simulink model "Md53StEnCtrl"  (R2018b)
settings: Solver=FixedStepDiscrete  StartTime=0.0  StopTime=10.0  FixedStep=0.01  RelTol=1e-3
undefined symbols (not defined in the file or in its folder): data, SecRwRtStBkReclnEn_Clear, SecRwRtStBkReclnEn_Set, ThdRwRtStBkReclnEn_Clear, ThdRwRtStBkReclnEn_Set, ThdRwRtStCshnFldEn_Clear, ThdRwRtStCshnFldEn_Set
libraries: simulink x1
settings Model: Creator=sn2xws  LastModifiedBy=sn2xws
settings Model: ModifiedHistory=|
  | 2024.6.24 V3.0.0 557模式流程V1.9
  | 2024.8.16 V3.0.1增加FirstTrig参数
  | 2024.8.20 V3.0.2 CshnFirstDone 时不调用电机
  | 2024.12.17 V3.0.3 BUG 962503 三排靠背与二排靠背应该一起动
settings DataIOCC: SaveFormat=StructureWithTime
settings OptimizationCC: DefaultParameterBehavior=Inlined  EnhancedBackFolding=on  PassReuseOutputArgsAs=Individual arguments  ZeroExternalMemoryAtStartup=off  ZeroInternalMemoryAtStartup=off  OptimizeBlockOrder=speed  DifferentSizesBufferReuse=on  OptimizationCustomize=off
settings DebuggingCC: ParameterTunabilityLossMsg=error
settings SFSimCC: MATLABDynamicMemAlloc=off
settings RTWCC: SystemTargetFile=autosar.tlc  GenCodeOnly=on  TemplateMakefile=ert_default_tmf  Description=AUTOSAR  GenerateReport=on  IncludeHyperlinkInReport=on  LaunchReport=on  GenerateTraceInfo=on  GenerateTraceReport=on  GenerateTraceReportSl=on  GenerateTraceReportSf=on  GenerateTraceReportEml=on
settings CodeAppCC: ForceParamTrailComments=on  IgnoreCustomStorageClasses=off  OperatorAnnotations=on  SimulinkDataObjDesc=on  SFDataObjDesc=on  InsertBlockDesc=on
settings STFCustomTargetCC: TargetLangStandard=C99 (ISO)  MultiwordLength=256  ParMdlRefBuildCompliant=on  CompOptLevelCompliant=on  IncludeMdlTerminateFcn=off  CombineOutputUpdateFcns=on  SuppressErrorStatus=on  ERTCustomFileBanners=on  SupportNonFinite=off  SupportComplex=off  SupportContinuousTime=off  SupportNonInlinedSFcns=off  RemoveResetFunc=on  MATLABClassNameForMDSCustomization=Simulink.SoftwareTarget.ERTCustomization  AutosarCompliant=on  UseToolchainInfoCompliant=on  LookupTableObjectStructAxisOrder=2,1,3,4,...  LUTObjectStructOrderEvenSpacing=Size,Table,Breakpoints  SystemTargetFile=autosar.tlc
settings ERTTargetCC: TargetLangStandard=C99 (ISO)  ConcurrentExecutionCompliant=off  IncludeMdlTerminateFcn=off  SuppressErrorStatus=on  SupportNonFinite=off  SupportComplex=off  ModelStepFunctionPrototypeControlCompliant=off  CPPClassGenCompliant=off  AutosarCompliant=on  LookupTableObjectStructAxisOrder=2,1,3,4,...  LUTObjectStructOrderEvenSpacing=Size,Table,Breakpoints  InlinedParameterPlacement=NonHierarchical  ERTCustomFileTemplate=example_file_process.tlc  ERTFilePackagingFormat=Compact

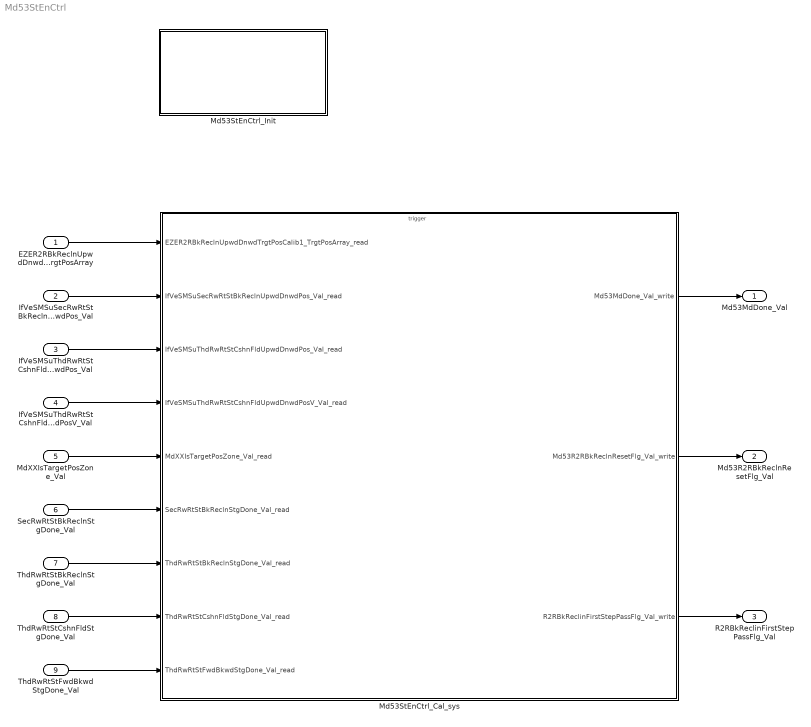
== system Md53StEnCtrl ==
  EZER2RBkReclnUpwdDnwdTrgtPosCalib1_TrgtPosArray : Inport  Description=|  OutDataTypeStr=uint16  PortDimensions=3
      | 0:Pos
      | 1:Max
      | 2:Min
  IfVeSMSuSecRwRtStBkReclnUpwdDnwdPos_Val : Inport  Port=2  OutDataTypeStr=uint16  PortDimensions=1
  IfVeSMSuThdRwRtStCshnFldUpwdDnwdPos_Val : Inport  Port=3  OutDataTypeStr=uint16  PortDimensions=1
  IfVeSMSuThdRwRtStCshnFldUpwdDnwdPosV_Val : Inport  Port=4  OutDataTypeStr=boolean  PortDimensions=1
  MdXXIsTargetPosZone_Val : Inport  Port=5  OutDataTypeStr=uint32  PortDimensions=1
  SecRwRtStBkReclnStgDone_Val : Inport  Port=6  OutDataTypeStr=boolean  PortDimensions=1
  ThdRwRtStBkReclnStgDone_Val : Inport  Port=7  OutDataTypeStr=boolean  PortDimensions=1
  ThdRwRtStCshnFldStgDone_Val : Inport  Port=8  OutDataTypeStr=boolean  PortDimensions=1
  ThdRwRtStFwdBkwdStgDone_Val : Inport  Port=9  OutDataTypeStr=boolean  PortDimensions=1
  Md53StEnCtrl_Cal_sys : Subsystem
  Md53StEnCtrl_Init : Subsystem
  Md53MdDone_Val : Outport  OutDataTypeStr=uint8  PortDimensions=1
  Md53R2RBkReclnResetFlg_Val : Outport  Port=2  OutDataTypeStr=boolean  PortDimensions=1
  R2RBkReclinFirstStepPassFlg_Val : Outport  Port=3  OutDataTypeStr=boolean  PortDimensions=1
  wires:
  EZER2RBkReclnUpwdDnwdTrgtPosCalib1_TrgtPosArray/1 -> Md53StEnCtrl_Cal_sys/1(EZER2RBkReclnUpwdDnwdTrgtPosCalib1_TrgtPosArray_read)
  IfVeSMSuSecRwRtStBkReclnUpwdDnwdPos_Val/1 -> Md53StEnCtrl_Cal_sys/2(IfVeSMSuSecRwRtStBkReclnUpwdDnwdPos_Val_read)
  IfVeSMSuThdRwRtStCshnFldUpwdDnwdPos_Val/1 -> Md53StEnCtrl_Cal_sys/3(IfVeSMSuThdRwRtStCshnFldUpwdDnwdPos_Val_read)
  IfVeSMSuThdRwRtStCshnFldUpwdDnwdPosV_Val/1 -> Md53StEnCtrl_Cal_sys/4(IfVeSMSuThdRwRtStCshnFldUpwdDnwdPosV_Val_read)
  MdXXIsTargetPosZone_Val/1 -> Md53StEnCtrl_Cal_sys/5(MdXXIsTargetPosZone_Val_read)
  SecRwRtStBkReclnStgDone_Val/1 -> Md53StEnCtrl_Cal_sys/6(SecRwRtStBkReclnStgDone_Val_read)
  ThdRwRtStBkReclnStgDone_Val/1 -> Md53StEnCtrl_Cal_sys/7(ThdRwRtStBkReclnStgDone_Val_read)
  ThdRwRtStCshnFldStgDone_Val/1 -> Md53StEnCtrl_Cal_sys/8(ThdRwRtStCshnFldStgDone_Val_read)
  ThdRwRtStFwdBkwdStgDone_Val/1 -> Md53StEnCtrl_Cal_sys/9(ThdRwRtStFwdBkwdStgDone_Val_read)
  Md53StEnCtrl_Cal_sys/1(Md53MdDone_Val_write) -> Md53MdDone_Val/1
  Md53StEnCtrl_Cal_sys/2(Md53R2RBkReclnResetFlg_Val_write) -> Md53R2RBkReclnResetFlg_Val/1
  Md53StEnCtrl_Cal_sys/3(R2RBkReclinFirstStepPassFlg_Val_write) -> R2RBkReclinFirstStepPassFlg_Val/1

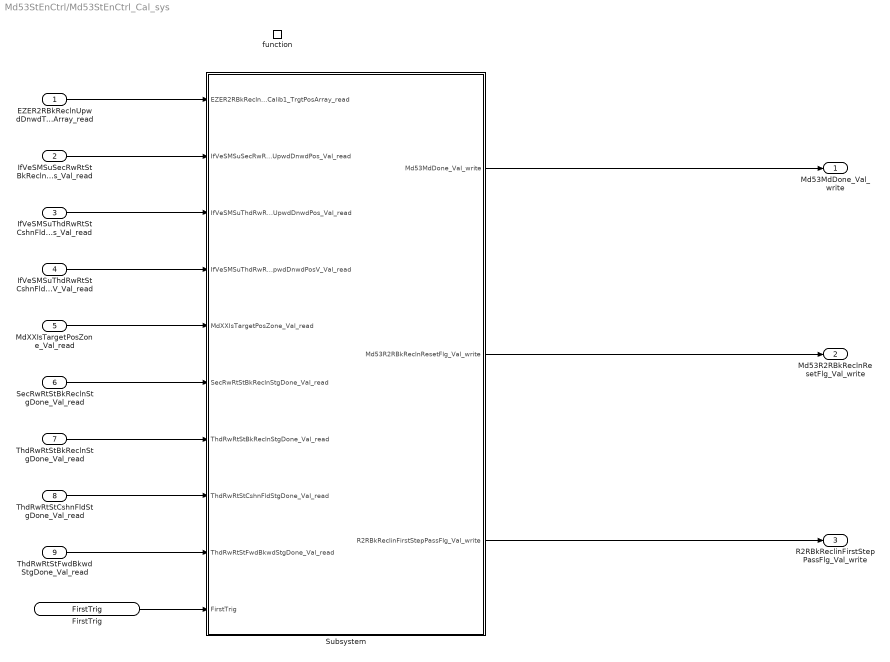
== system Md53StEnCtrl/Md53StEnCtrl_Cal_sys ==
  EZER2RBkReclnUpwdDnwdTrgtPosCalib1_TrgtPosArray_read : Inport
  IfVeSMSuSecRwRtStBkReclnUpwdDnwdPos_Val_read : Inport  Port=2
  IfVeSMSuThdRwRtStCshnFldUpwdDnwdPos_Val_read : Inport  Port=3
  IfVeSMSuThdRwRtStCshnFldUpwdDnwdPosV_Val_read : Inport  Port=4
  MdXXIsTargetPosZone_Val_read : Inport  Port=5
  SecRwRtStBkReclnStgDone_Val_read : Inport  Port=6
  ThdRwRtStBkReclnStgDone_Val_read : Inport  Port=7
  ThdRwRtStCshnFldStgDone_Val_read : Inport  Port=8
  ThdRwRtStFwdBkwdStgDone_Val_read : Inport  Port=9
  function : TriggerPort  TriggerType=function-call  IsSimulinkFunction=on  FunctionName=Md53StEnCtrl_Cal  VariantControl=(inherit)
  Subsystem : Subsystem
  FirstTrig : ArgIn  OutDataTypeStr=boolean  ArgumentName=FirstTrig
  Md53MdDone_Val_write : Outport
      settings: EnsureOutportIsVirtual=on
  Md53R2RBkReclnResetFlg_Val_write : Outport  Port=2
      settings: EnsureOutportIsVirtual=on
  R2RBkReclinFirstStepPassFlg_Val_write : Outport  Port=3
      settings: EnsureOutportIsVirtual=on
  wires:
  EZER2RBkReclnUpwdDnwdTrgtPosCalib1_TrgtPosArray_read/1 -> Subsystem/1(EZER2RBkReclnUpwdDnwdTrgtPosCalib1_TrgtPosArray_read)
  IfVeSMSuSecRwRtStBkReclnUpwdDnwdPos_Val_read/1 -> Subsystem/2(IfVeSMSuSecRwRtStBkReclnUpwdDnwdPos_Val_read)
  IfVeSMSuThdRwRtStCshnFldUpwdDnwdPos_Val_read/1 -> Subsystem/3(IfVeSMSuThdRwRtStCshnFldUpwdDnwdPos_Val_read)
  IfVeSMSuThdRwRtStCshnFldUpwdDnwdPosV_Val_read/1 -> Subsystem/4(IfVeSMSuThdRwRtStCshnFldUpwdDnwdPosV_Val_read)
  MdXXIsTargetPosZone_Val_read/1 -> Subsystem/5(MdXXIsTargetPosZone_Val_read)
  SecRwRtStBkReclnStgDone_Val_read/1 -> Subsystem/6(SecRwRtStBkReclnStgDone_Val_read)
  ThdRwRtStBkReclnStgDone_Val_read/1 -> Subsystem/7(ThdRwRtStBkReclnStgDone_Val_read)
  ThdRwRtStCshnFldStgDone_Val_read/1 -> Subsystem/8(ThdRwRtStCshnFldStgDone_Val_read)
  ThdRwRtStFwdBkwdStgDone_Val_read/1 -> Subsystem/9(ThdRwRtStFwdBkwdStgDone_Val_read)
  Subsystem/1(Md53MdDone_Val_write) -> Md53MdDone_Val_write/1
  Subsystem/2(Md53R2RBkReclnResetFlg_Val_write) -> Md53R2RBkReclnResetFlg_Val_write/1
  Subsystem/3(R2RBkReclinFirstStepPassFlg_Val_write) -> R2RBkReclinFirstStepPassFlg_Val_write/1
  FirstTrig/1 -> Subsystem/10(FirstTrig)

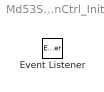
== system Md53StEnCtrl/Md53StEnCtrl_Init ==
  Event Listener : EventListener  EventName=reset

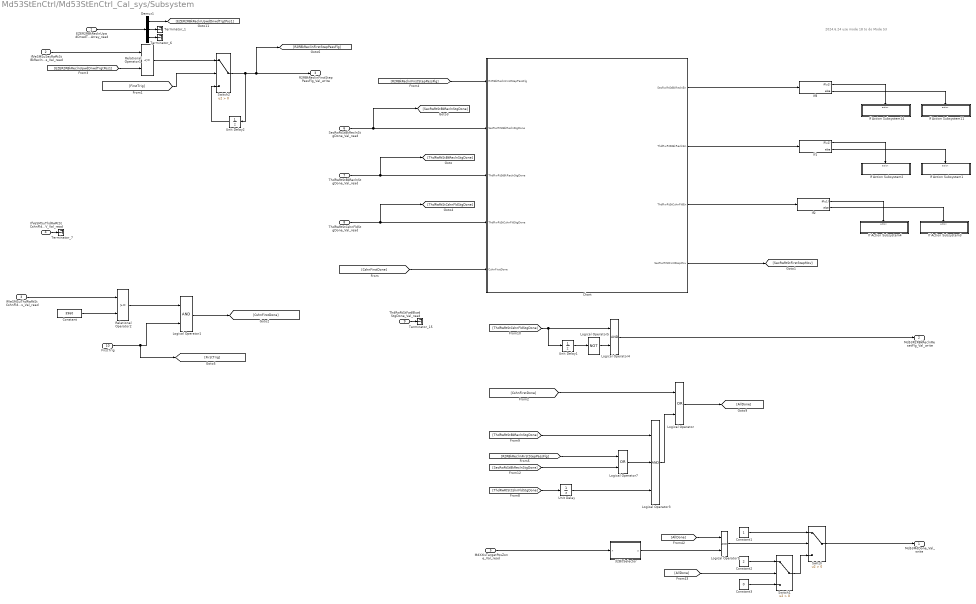
== system Md53StEnCtrl/Md53StEnCtrl_Cal_sys/Subsystem ==
  note: 2024.6.24 use mode 18 to do Mode 53
  EZER2RBkReclnUpwdDnwdTrgtPosCalib1_TrgtPosArray_read : Inport
  IfVeSMSuSecRwRtStBkReclnUpwdDnwdPos_Val_read : Inport  Port=2
  IfVeSMSuThdRwRtStCshnFldUpwdDnwdPos_Val_read : Inport  Port=3
  IfVeSMSuThdRwRtStCshnFldUpwdDnwdPosV_Val_read : Inport  Port=4
  MdXXIsTargetPosZone_Val_read : Inport  Port=5
  SecRwRtStBkReclnStgDone_Val_read : Inport  Port=6
  ThdRwRtStBkReclnStgDone_Val_read : Inport  Port=7
  ThdRwRtStCshnFldStgDone_Val_read : Inport  Port=8
  ThdRwRtStFwdBkwdStgDone_Val_read : Inport  Port=9
  FirstTrig : Inport  Port=10
  32BitSelector : Subsystem  mask(32 Bit Selector){BitNum=17}
      mask prompts: BitNum "Select Bit Number"
      mask help: Allows selection of a particular bit (0-31) out of a packed word up to 32 bits long. Output will be true if the bit number selected via the mask parameter is equal to one.
      mask TypeOptions BitNum: 0 | 1 | 2 | 3 | 4 | 5 | 6 | 7 | 8 | 9 | 10 | 11 | 12 | 13 | 14 | 15 | 16 | 17 | 18 | 19 | 20 | 21 | 22 | 23 | 24 | 25 | 26 | 27 | 28 | 29 | 30 | 31
      mask Display:
      | text(0.5, 0.8,'BIT','horizontalAlignment','center')
      | text(0.5, 0.5,'SELECTOR','horizontalAlignment','center')
      | text(0.5, 0.2,['-- Bit ',char(get_param(gcb,'BitNum')),' --'],'horizontalAlignment','center')
  Chart : Stateflow chart  TreatAsAtomicUnit=on
  Constant : Constant  Value=3960  OutDataTypeStr=uint16
  Constant1 : Constant  OutDataTypeStr=uint8
  Constant2 : Constant  Value=2  OutDataTypeStr=uint8
  Constant3 : Constant  Value=0  OutDataTypeStr=uint8
  Demux1 : Demux  Outputs=3
  If Action Subsystem1 : Subsystem  TreatAsAtomicUnit=on
  If Action Subsystem11 : Subsystem  TreatAsAtomicUnit=on
  If Action Subsystem14 : Subsystem  TreatAsAtomicUnit=on
  If Action Subsystem2 : Subsystem  TreatAsAtomicUnit=on
  If Action Subsystem3 : Subsystem  TreatAsAtomicUnit=on
  If Action Subsystem4 : Subsystem  TreatAsAtomicUnit=on
  If1 : If  IfExpression=u1
  If2 : If  IfExpression=u1
  If8 : If  IfExpression=u1
  Logical Operator : Logic  Operator=OR  AllPortsSameDT=off  OutDataTypeStr=boolean
  Logical Operator1 : Logic  AllPortsSameDT=off  OutDataTypeStr=boolean
  Logical Operator3 : Logic  Inputs=3  AllPortsSameDT=off  OutDataTypeStr=boolean
  Logical Operator4 : Logic  AllPortsSameDT=off  OutDataTypeStr=boolean
  Logical Operator5 : Logic  Operator=NOT  AllPortsSameDT=off  OutDataTypeStr=boolean
  Logical Operator7 : Logic  Operator=OR  AllPortsSameDT=off  OutDataTypeStr=boolean
  Logical Operator9 : Logic  AllPortsSameDT=off  OutDataTypeStr=boolean
  Relational Operator1 : RelationalOperator  Operator=<=  OutDataTypeStr=boolean  RndMeth=Simplest
  Relational Operator2 : RelationalOperator  OutDataTypeStr=boolean  RndMeth=Simplest
  Switch : Switch  Criteria=u2 > Threshold
  Switch1 : Switch  Criteria=u2 > Threshold
  Switch2 : Switch  Criteria=u2 > Threshold
  Terminator_{1,6..7,15} (4 alike) : Terminator
  Unit Delay : UnitDelay  SampleTime=-1
  Unit Delay1 : UnitDelay  SampleTime=-1
  Unit Delay2 : UnitDelay  SampleTime=-1
  Md53MdDone_Val_write : Outport
      settings: EnsureOutportIsVirtual=on
  Md53R2RBkReclnResetFlg_Val_write : Outport  Port=2
      settings: EnsureOutportIsVirtual=on
  R2RBkReclinFirstStepPassFlg_Val_write : Outport  Port=3
      settings: EnsureOutportIsVirtual=on
  wires:
  IfVeSMSuThdRwRtStCshnFldUpwdDnwdPosV_Val_read/1 -> Terminator_7/1
  ThdRwRtStCshnFldStgDone_Val_read/1 -> [ThdRwRtStCshnFldStgDone], Chart/4(ThdRwRtStCshnFldStgDone)
  ThdRwRtStBkReclnStgDone_Val_read/1 -> [ThdRwRtStBkReclnStgDone], Chart/3(ThdRwRtStBkReclnStgDone)
  ThdRwRtStFwdBkwdStgDone_Val_read/1 -> Terminator_15/1
  SecRwRtStBkReclnStgDone_Val_read/1 -> [SecRwRtStBkReclnStgDone], Chart/2(SecRwRtStBkReclnStgDone)
  Switch/1 -> Md53MdDone_Val_write/1
  Logical Operator4/1 -> Md53R2RBkReclnResetFlg_Val_write/1
  [AllDone] -> Logical Operator9/1
  Logical Operator9/1 -> Switch/2
  Switch1/1 -> Switch/3
  Constant1/1 -> Switch/1
  32BitSelector/1(y) -> Logical Operator9/2
  Constant2/1 -> Switch1/1
  [AllDone] -> Switch1/2
  MdXXIsTargetPosZone_Val_read/1 -> 32BitSelector/1(x)
  Constant3/1 -> Switch1/3
  [R2RBkReclinFirstStepPassFlg] -> Logical Operator7/1
  Logical Operator/1 -> [AllDone]
  [SecRwRtStBkReclnStgDone] -> Logical Operator7/2
  [ThdRwRtStBkReclnStgDone] -> Logical Operator3/1
  Logical Operator3/1 -> Logical Operator/2
  [ThdRwRtStCshnFldStgDone] -> Unit Delay/1
  Unit Delay/1 -> Logical Operator3/3
  Logical Operator7/1 -> Logical Operator3/2
  [CshnFirstDone] -> Logical Operator/1
  Logical Operator5/1 -> Logical Operator4/2
  [ThdRwRtStCshnFldStgDone] -> Unit Delay1/1, Logical Operator4/1
  Unit Delay1/1 -> Logical Operator5/1
  Constant/1 -> Relational Operator2/2
  IfVeSMSuThdRwRtStCshnFldUpwdDnwdPos_Val_read/1 -> Relational Operator2/1
  [CshnFirstDone] -> Chart/5(CshnFirstDone)
  Chart/4(SecRwRtStFirstStepMov) -> [SecRwRtStFirstStepMov]
  Demux1/1 -> [EZER2RBkReclnUpwdDnwdTrgtPos1]
  Demux1/3 -> Terminator_6/1
  Demux1/2 -> Terminator_1/1
  EZER2RBkReclnUpwdDnwdTrgtPosCalib1_TrgtPosArray_read/1 -> Demux1/1
  [EZER2RBkReclnUpwdDnwdTrgtPos1] -> Relational Operator1/2
  IfVeSMSuSecRwRtStBkReclnUpwdDnwdPos_Val_read/1 -> Relational Operator1/1
  Chart/1(SecRwRtStBkReclnEn) -> If8/1
  If8/2 -> If Action Subsystem11/Action
  If8/1 -> If Action Subsystem14/Action
  If1/1 -> If Action Subsystem2/Action
  If1/2 -> If Action Subsystem1/Action
  Chart/2(ThdRwRtStBkReclnEn) -> If1/1
  Chart/3(ThdRwRtStCshnFldEn) -> If2/1
  If2/2 -> If Action Subsystem3/Action
  If2/1 -> If Action Subsystem4/Action
  Logical Operator1/1 -> [CshnFirstDone]
  Relational Operator2/1 -> Logical Operator1/1
  FirstTrig/1 -> [FirstTrig], Logical Operator1/2
  [FirstTrig] -> Switch2/2
  Relational Operator1/1 -> Switch2/1
  Switch2/1 -> [R2RBkReclinFirstStepPassFlg], R2RBkReclinFirstStepPassFlg_Val_write/1, Unit Delay2/1
  Unit Delay2/1 -> Switch2/3
  [R2RBkReclinFirstStepPassFlg] -> Chart/1(R2RBkReclinFirstStepPassFlg)

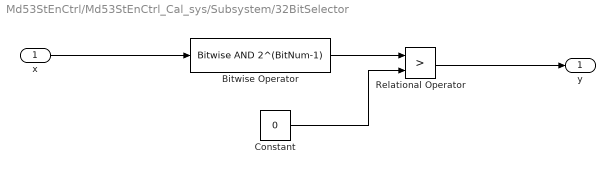
== system Md53StEnCtrl/Md53StEnCtrl_Cal_sys/Subsystem/32BitSelector ==
  x : Inport
  Bitwise Operator : simulink/Logic and Bit Operations/Bitwise Operator  logicop=AND  UseBitMask=on  BitMask=2^(BitNum-1)  BitMaskRealWorld=Stored Integer
  Constant : Constant  Value=0  OutDataTypeStr=uint32
  Relational Operator : RelationalOperator  Operator=>  OutDataTypeStr=boolean  RndMeth=Simplest
  y : Outport
  wires:
  Relational Operator/1 -> y/1
  Constant/1 -> Relational Operator/2
  x/1 -> Bitwise Operator/1
  Bitwise Operator/1 -> Relational Operator/1

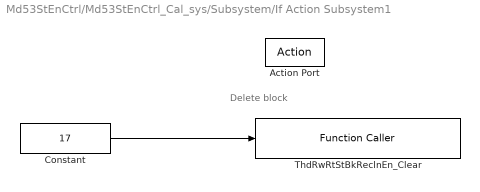
== system Md53StEnCtrl/Md53StEnCtrl_Cal_sys/Subsystem/If Action Subsystem1 ==
  note: Delete block
  Action Port : ActionPort  ActionType=else
  Constant : Constant  Value=17  OutDataTypeStr=uint8
  ThdRwRtStBkReclnEn_Clear : FunctionCaller  FunctionPrototype=ThdRwRtStBkReclnEn_Clear(data)  InputArgumentSpecifications=uint8(1)
  wires:
  Constant/1 -> ThdRwRtStBkReclnEn_Clear/1

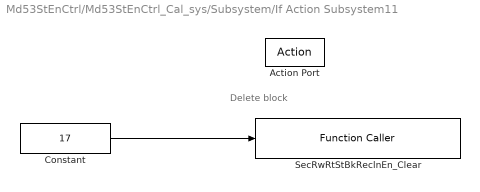
== system Md53StEnCtrl/Md53StEnCtrl_Cal_sys/Subsystem/If Action Subsystem11 ==
  note: Delete block
  Action Port : ActionPort  ActionType=else
  Constant : Constant  Value=17  OutDataTypeStr=uint8
  SecRwRtStBkReclnEn_Clear : FunctionCaller  FunctionPrototype=SecRwRtStBkReclnEn_Clear(data)  InputArgumentSpecifications=uint8(1)
  wires:
  Constant/1 -> SecRwRtStBkReclnEn_Clear/1

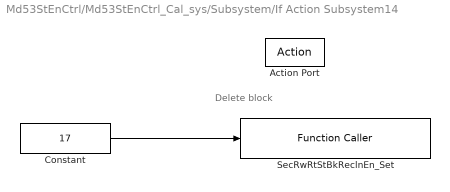
== system Md53StEnCtrl/Md53StEnCtrl_Cal_sys/Subsystem/If Action Subsystem14 ==
  note: Delete block
  Action Port : ActionPort  ActionType=then
  Constant : Constant  Value=17  OutDataTypeStr=uint8
  SecRwRtStBkReclnEn_Set : FunctionCaller  FunctionPrototype=SecRwRtStBkReclnEn_Set(data)  InputArgumentSpecifications=uint8(1)
  wires:
  Constant/1 -> SecRwRtStBkReclnEn_Set/1

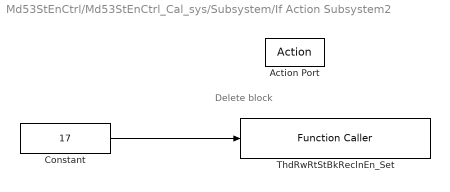
== system Md53StEnCtrl/Md53StEnCtrl_Cal_sys/Subsystem/If Action Subsystem2 ==
  note: Delete block
  Action Port : ActionPort  ActionType=then
  Constant : Constant  Value=17  OutDataTypeStr=uint8
  ThdRwRtStBkReclnEn_Set : FunctionCaller  FunctionPrototype=ThdRwRtStBkReclnEn_Set(data)  InputArgumentSpecifications=uint8(1)
  wires:
  Constant/1 -> ThdRwRtStBkReclnEn_Set/1

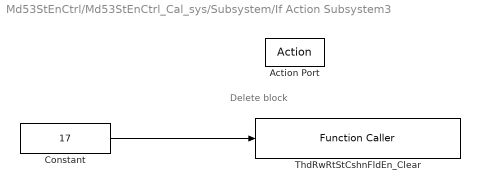
== system Md53StEnCtrl/Md53StEnCtrl_Cal_sys/Subsystem/If Action Subsystem3 ==
  note: Delete block
  Action Port : ActionPort  ActionType=else
  Constant : Constant  Value=17  OutDataTypeStr=uint8
  ThdRwRtStCshnFldEn_Clear : FunctionCaller  FunctionPrototype=ThdRwRtStCshnFldEn_Clear(data)  InputArgumentSpecifications=uint8(1)
  wires:
  Constant/1 -> ThdRwRtStCshnFldEn_Clear/1

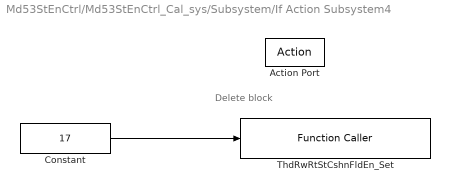
== system Md53StEnCtrl/Md53StEnCtrl_Cal_sys/Subsystem/If Action Subsystem4 ==
  note: Delete block
  Action Port : ActionPort  ActionType=then
  Constant : Constant  Value=17  OutDataTypeStr=uint8
  ThdRwRtStCshnFldEn_Set : FunctionCaller  FunctionPrototype=ThdRwRtStCshnFldEn_Set(data)  InputArgumentSpecifications=uint8(1)
  wires:
  Constant/1 -> ThdRwRtStCshnFldEn_Set/1

== stateflow chart Md53StEnCtrl/Md53StEnCtrl_Cal_sys/Subsystem/Chart ==
  (default) -> (junction 22) : {
      | SecRwRtStBkReclnEn = 0;
      | ThdRwRtStCshnFldEn = 0;
      | ThdRwRtStBkReclnEn = 0;
      | }
  (junction 22) -> (junction 83) [order 1] : [CshnFirstDone]
  (junction 22) -> (junction 25) [order 2]
  (junction 83) -> (junction 85)
  (junction 25) -> (junction 27) [order 1] : [R2RBkReclinFirstStepPassFlg ||SecRwRtStBkReclnStgDone]
  (junction 25) -> (junction 31) [order 2] : {
      | SecRwRtStBkReclnEn = 1;
      | }
  (junction 27) -> (junction 29)
  (junction 29) -> (junction 31)
  (junction 31) -> (junction 34)
  (junction 34) -> (junction 36) [order 1] : [(R2RBkReclinFirstStepPassFlg ||SecRwRtStBkReclnStgDone)]
  (junction 36) -> (junction 43) [order 1] : [ThdRwRtStCshnFldStgDone]
  (junction 34) -> (junction 75) [order 2]
  (junction 36) -> (junction 38) [order 2] : {ThdRwRtStCshnFldEn = 1;}
  (junction 43) -> (junction 66)
  (junction 38) -> (junction 75)
  (junction 66) -> (junction 38)
  (junction 75) -> (junction 78)
  (junction 78) -> (junction 94) [order 1] : [ThdRwRtStCshnFldStgDone]
  (junction 94) -> (junction 95) [order 1] : [ThdRwRtStBkReclnStgDone]
  (junction 78) -> (junction 97) [order 2]
  (junction 94) -> (junction 96) [order 2] : {
      | ThdRwRtStBkReclnEn =1;
      | }
  (junction 95) -> (junction 88)
  (junction 96) -> (junction 97)
  (junction 88) -> (junction 96)
  (junction 85) -> (junction 88)
  (junction 97) -> (junction 100)
  data: R2RBkReclinFirstStepPassFlg input; SecRwRtStBkReclnStgDone input; ThdRwRtStBkReclnStgDone input; ThdRwRtStCshnFldStgDone input; SecRwRtStBkReclnEn output boolean; ThdRwRtStBkReclnEn output boolean; ThdRwRtStCshnFldEn output boolean; CshnFirstDone input; SecRwRtStFirstStepMov output boolean
